simulink model "HILBackEnd"  (R2024a)
settings: Solver=FixedStepAuto  StartTime=0.0  StopTime=inf  RelTol=1e-3
undefined symbols (not defined in the file or in its folder): f
libraries: instrumentlib x2
settings Model: Creator=natha  LastModifiedBy=natha

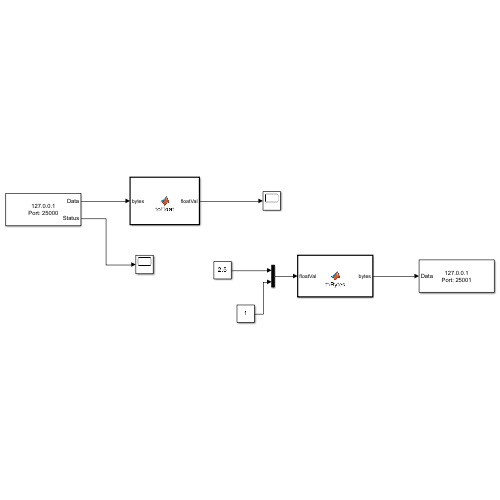
[thumbnail: Simulink's stored preview of the top-level diagram]
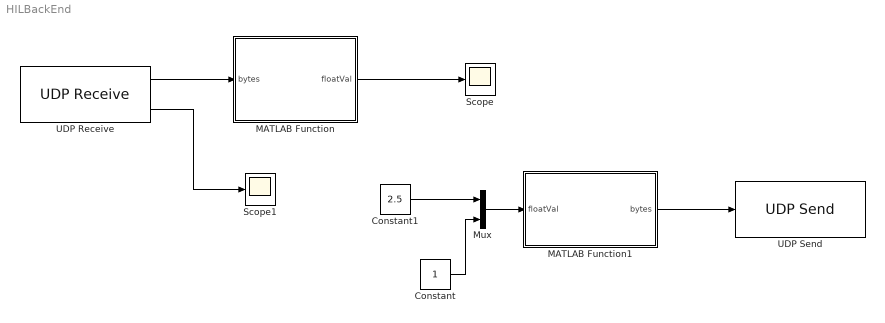
== system HILBackEnd ==
  Constant : Constant
  Constant1 : Constant  Value=2.5
  MATLAB Function : MATLAB Function  TreatAsAtomicUnit=on
  MATLAB Function1 : MATLAB Function  TreatAsAtomicUnit=on
  Mux : Mux  Inputs=2
  Scope : Scope
  Scope1 : Scope
  UDP Receive : instrumentlib/UDP Receive  LocalAddress=127.0.0.1  LocalPort=25000  EnablePortSharing=off  Host=localhost  Port=25001  GetLatestData=on  DataSize=[ 1, 16 ]  DataType=uint8  ASCIIFormatting=%f,  Terminator=LF  CustomTerminator=10  ByteOrder=big-endian  EnableBlockingMode=off  Timeout=10  SampleTime=0.01  SimulateUsing=Interpreted execution
  UDP Send : instrumentlib/UDP Send  Host=127.0.0.1  Port=25001  LocalAddress=127.0.0.1  LocalPort=25000  EnablePortSharing=off  OutputDatagramPacketSize=32  ByteOrder=big-endian  EnableBlockingMode=off  SimulateUsing=Interpreted execution
  wires:
  UDP Receive/1 -> MATLAB Function/1(bytes)
  UDP Receive/2 -> Scope1/1
  MATLAB Function/1(floatVal) -> Scope/1
  MATLAB Function1/1(bytes) -> UDP Send/1
  Mux/1 -> MATLAB Function1/1(floatVal)
  Constant1/1 -> Mux/1
  Constant/1 -> Mux/2

== matlab function HILBackEnd/MATLAB Function ==
  data: bytes input; floatVal output
function floatVal = toFloat(bytes)
%constants-------------
numFloats = 2;
%----------------------
floatVal = zeros(1,numFloats,'double');
if(length(bytes) == 8*numFloats)
    floatVal = typecast(uint8(bytes), 'double');
end
end

== matlab function HILBackEnd/MATLAB Function1 ==
  data: floatVal input; bytes output uint8 size=[1 16]
function bytes = toBytes(floatVal)
%constants-------------
numFloats = 2;
%----------------------
bytes = zeros(1,numFloats*8,'uint8');
if(length(floatVal) == numFloats)
    bytes = typecast(double(floatVal), 'uint8')';
end
end
